simulink model "Battery_Module_Design_Grouped"  (R2021b)
settings: Solver=ode23t  StartTime=0.0  StopTime=36000  MaxStep=0.05  RelTol=1e-3  AbsTol=1e-3
undefined symbols (not defined in the file): batteryCurrent
libraries: fl_lib x5, nesl_utility x4, batteryModule_lib x1
Description:
  | Battery Pack Thermal Management
  | 
  | Copyright 2020-2021 The MathWorks, Inc.
settings Model: Creator=vikrants  LastModifiedBy=smiller
settings SolverCC: AutoScaleAbsTol=off  AlgebraicLoopSolver=TrustRegion
settings DataIOCC: ReturnWorkspaceOutputs=off  SignalLoggingName=logsout_Battery_Module_Design_Grouped
settings DebuggingCC: SymbolicDimsDataTypeCodeGenerationDiagnostic=none  SFMachineParentedDataDiag=warning
settings SFSimCC: CustomCodeUndefinedFunction=UseInterfaceOnly
settings SimscapeCC: SimscapeLogType=all  SimscapeLogSimulationStatistics=on  SimscapeLogName=simlog_Battery_Module_Design_Grouped  SimscapeLogDataHistory=250000

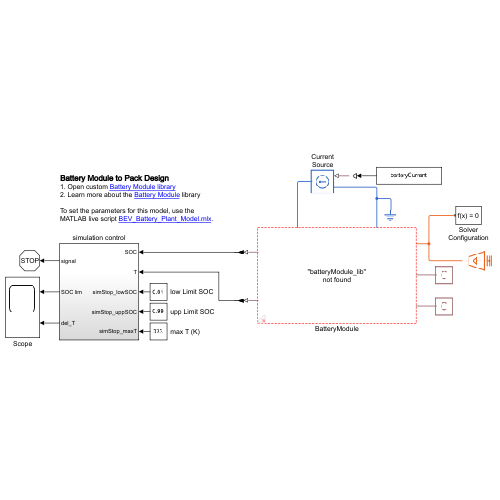
[thumbnail: Simulink's stored preview of the top-level diagram]
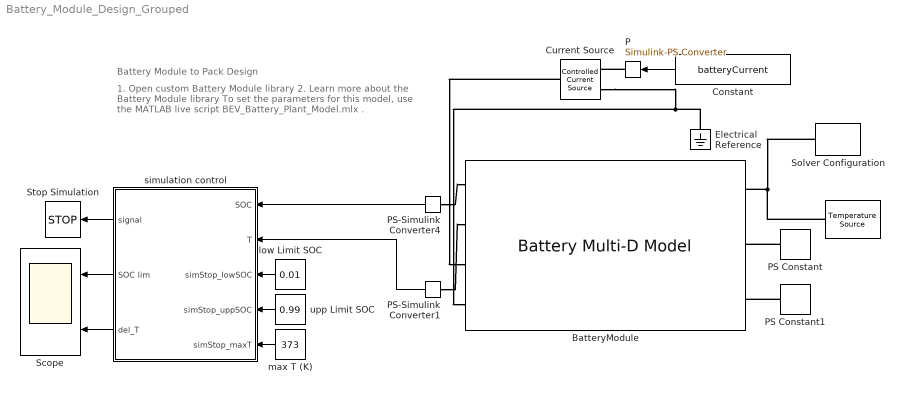
== system Battery_Module_Design_Grouped ==
  note: 1. Open custom Battery Module library
      | 2. Learn more about the Battery Module library
      |
      | To set the parameters for this model, use the
      | MATLAB live script BEV_Battery_Plant_Model.mlx .
  note: Battery Module to Pack Design
  " " : fl_lib/Thermal/Thermal Sources/Temperature Source  temperature=ambientTemp K
  BatteryModule : batteryModule_lib/Battery Multi-D Model  modelComplexity=batteryModule.batteryAbstractionLevel.grouped  thermalManagement=batteryModule.batteryCoolingSystem.thermalPort  thermal_moduleBottom=batteryModule.batteryThermalPortSelection.thermalLUT  thermal_moduleTop=batteryModule.batteryThermalPortSelection.convectionBC  thermal_moduleLeft=batteryModule.batteryThermalPortSelection.convectionBC  thermal_moduleRight=batteryModule.batteryThermalPortSelection.convectionBC  thermal_modulePos=batteryModule.batteryThermalPortSelection.convectionBC  thermal_moduleNeg=batteryModule.batteryThermalPortSelection.convectionBC  Ns=battery_Ns  Np=battery_Np  cellTypeSelection=batteryModule.batteryTypeSelection.pouch  cellHeight=battery_cellH m  cellWidth=battery_cellW m  cellThickness=battery_cellT m  cellDiameter=0.018 m  cellCylinLine=3  moduleExternalR=battery_extR Ohm  LUTpointsTemp=battery_vecT K  LUTpointsSOC=battery_vecSOC  cellAHvector=battery_vecAhr hr*A  moduleCellAHpercentVar=battery_varAhr  cellThermalMass=battery_thermalMass J/K  cellThermalCond=battery_thermalK_thru W/(m*K)  cellThermalCond_inPlane=battery_thermalK_in W/(m*K)  cellHeatTrCoeff=1 W/(m^2 * K)  htc_bottom=1 W/(m^2 * K)  htc_top=battery_sidesHTC W/(m^2 * K)  htc_right=battery_sidesHTC W/(m^2 * K)  htc_left=battery_sidesHTC W/(m^2 * K)  htc_pos=battery_sidesHTC W/(m^2 * K)  htc_neg=battery_sidesHTC W/(m^2 * K)  cellTemp=battery_iniT K  cellSOC=battery_iniSOC  LUTpointsFlowrate_b=vec_coolant_F kg/s  LUTpointsTemp_b=vec_coolant_T K  LUTpointsFlowrate_t=[.01, .02, .03, .04, .05, .06] kg/s  LUTpointsTemp_t=[273.15, 298.15, 323.15] K  LUTpointsFlowrate_r=[.01, .02, .03, .04, .05, .06] kg/s  LUTpointsTemp_r=[273.15, 298.15, 323.15] K  LUTpointsFlowrate_l=[.01, .02, .03, .04, .05, .06] kg/s  LUTpointsTemp_l=[273.15, 298.15, 323.15] K  LUTpointsFlowrate_p=[.01, .02, .03, .04, .05, .06] kg/s  LUTpointsTemp_p=[273.15, 298.15, 323.15] K  LUTpointsFlowrate_n=[.01, .02, .03, .04, .05, .06] kg/s  LUTpointsTemp_n=[273.15, 298.15, 323.15] K  moduleCooling_b=mat_cellQ W/K  moduleCooling_t=zeros(3, 6, 10) W/K  moduleCooling_r=zeros(3, 6, 10) W/K  moduleCooling_l=zeros(3, 6, 10) W/K  moduleCooling_p=zeros(3, 6, 10) W/K  moduleCooling_n=zeros(3, 6, 10) W/K  moduleExtHeat=battery_extHeat W  moduleCellBalancing=batteryModule.batteryCellBalancing.none  passiveShuntR=50 Ohm  passiveSWclosedR=0.01 Ohm  passiveSWopenCond=1e-8 1/Ohm  passiveSWthreshold=0.5  prm_dir=ee.enum.battery.prm_dir.noCurrentDirectionality  V0_mat=battery_V0 V  R0_mat=battery_R0 Ohm  R0_dis_mat=[.03, .015, .002; .04, .017, .008; .039, .012, .006; .027, .013, .021] Ohm  R0_ch_mat=[.03, .015, .002; .04, .017, .008; .039, .012, .006; .027, .013, .021] Ohm  moduleCellR0PercentVar=battery_varR0  prm_leak=ee.enum.battery.prm_leak.disabled  Rleak_vec=[8000, 7000, 6000] Ohm  moduleCellLeakPercentVar=ones(1, 10)  extrapolation_option=ee.enum.extrapolation.nearest  prm_dyn=ee.enum.battery.prm_dyn.rc2  R1_mat=battery_R1 Ohm  tau1_mat=battery_Tau1 s  R2_mat=battery_R2 Ohm  tau2_mat=battery_Tau2 s  R3_mat=[.014, .382, .407; .028, .006, .007; .014, .007, .006; .333, .956, .912] Ohm  tau3_mat=[1, 44, 5644; 11, 24, 506; 2, 14, 330; 3310, 13419, 30216] s  R4_mat=[.014, .382, .407; .028, .006, .007; .014, .007, .006; .333, .956, .912] Ohm  tau4_mat=[1, 44, 5644; 11, 24, 506; 2, 14, 330; 3310, 13419, 30216] s  R5_mat=[.014, .382, .407; .028, .006, .007; .014, .007, .006; .333, .956, .912] Ohm  tau5_mat=[1, 44, 5644; 11, 24, 506; 2, 14, 330; 3310, 13419, 30216] s  prm_fade=ee.enum.battery.prm_fade.equations  N0=100  dV0=0  dR0=0  dAH=0  dRleak=0  dR1=0  dR2=0  dR3=0  dR4=0  dR5=0  N0vec=[100, 200, 300]  Tfadevec=[298.15, 323.15] K  dV0vec=[0, 0, 0]  dR0vec=[0, 0, 0]  dAHvec=[0, 0, 0]  dRleakvec=[0, 0, 0]  dR1vec=[0, 0, 0]  dR2vec=[0, 0, 0]  dR3vec=[0, 0, 0]  dR4vec=[0, 0, 0]  dR5vec=[0, 0, 0]  dV0mat=[0, 0; 0, 0; 0, 0]  dR0mat=[0, 0; 0, 0; 0, 0]  dAHmat=[0, 0; 0, 0; 0, 0]  dRleakmat=[0, 0; 0, 0; 0, 0]  dR1mat=[0, 0; 0, 0; 0, 0]  dR2mat=[0, 0; 0, 0; 0, 0]  dR3mat=[0, 0; 0, 0; 0, 0]  dR4mat=[0, 0; 0, 0; 0, 0]  dR5mat=[0, 0; 0, 0; 0, 0]
      settings: InternalSimscapePortConfiguration="{\"Bottom\":[],\"Left\":[{\"id\":\"outputCellSOC\",\"label\":\"SOC\",\"type\":\"output\"},{\"id\":\"outputCellTemp\",\"label\":\"Temp\",\"type\":\"output\"}],\"Right\":[{\"id\":\"H\",\"label\":\"Amb\",\"type\":\"foundation.thermal.thermal\"},{\"id\":\"frac_b\",\"label\":\"FlwR\",\"type\":\"input\"},{\"id\":\"delT_b\",\"label\":\"FlwT\",\"type\":\"input\"}],\"Top\":[{\"id\":\"p\",\"label\":\"pos\",\"type\":\"foundation.electrical.electrical\"},{\"id\":\"n\",\"label\":\"neg\",\"type\":\"foundation.electrical.electrical\"}]}"
  Constant : Constant  Value=batteryCurrent
  Current Source : fl_lib/Electrical/Electrical Sources/Controlled Current Source
  Electrical Reference : fl_lib/Electrical/Electrical Elements/Electrical Reference
  P : nesl_utility/Simulink-PS Converter  PhysicalDomain=network_engine_domain  SubClassName=ps_input  LeftPortType=input  RightPortType=output  PseudoPeriodic=off  Frequencies=[]  NoiseDistribution=none  NoiseParameters=[]  Unit=A  AffineConversion=off  FilteringAndDerivatives=provide  SimscapeFilterOrder=1  InputFilterTimeConstant=0.001  UdotUserProvided=0
      settings: SourceProductName=Utilities
  PS Constant : fl_lib/Physical Signals/Sources/PS Constant  constant=FlwR
  PS Constant1 : fl_lib/Physical Signals/Sources/PS Constant  constant=FlwT K
  PS-Simulink Converter1 : nesl_utility/PS-Simulink Converter  PhysicalDomain=network_engine_domain  SubClassName=ps_output  LeftPortType=input  RightPortType=output  PseudoPeriodic=off  Frequencies=[]  Unit=K  AffineConversion=on
      settings: SourceProductBaseCode=PW,SS
  PS-Simulink Converter4 : nesl_utility/PS-Simulink Converter  PhysicalDomain=network_engine_domain  SubClassName=ps_output  LeftPortType=input  RightPortType=output  PseudoPeriodic=off  Frequencies=[]  Unit=1  AffineConversion=on
      settings: SourceProductBaseCode=PW,SS
  Scope : Scope  NumInputPorts=2
  Solver Configuration : nesl_utility/Solver Configuration  PhysicalDomain=network_engine_domain  SubClassName=solver  LeftPortType=input  RightPortType=generic  Tones=[]  Harmonics=[]  SimulateNoise=off  Profile=off  UseLocalSampling=off  EnableSwitchedLinearOptims=on  FrequencyDomain=off  UseCCode=off  RelTol=0.001  AbsTol=1e-06  MinStep=1e-09  ToWorkspace=off  RevertToSquareIcSolve=off  NumHomotopyIterations=100  PhasorMode=off  PhasorModeNumHarmonics=1  DoDC=off  ResidualTolerance=1e-09  UseLocalSolver=off  LocalSolverChoice=NE_BACKWARD_EULER_ADVANCER  LocalSolverSampleTime=0.001  DoFixedCost=off  MaxNonlinIter=3  MaxModeIter=2  ComputeImpulses=off  ImpulseIterations=2  LinearAlgebra=auto  EquationFormulation=NE_TIME_EF  DelaysMemoryBudget=1024  AutomaticFiltering=on  FilteringTimeConstant=0.001  PartitionStorageMethod=AS_NEEDED  PartitionMemoryBudget=1024  PartitionMethod=ROBUST
      settings: SourceProductName=Utilities
  Stop Simulation : Stop
  low Limit SOC : Constant  Value=0.01
  max T (K) : Constant  Value=373
  simulation control : Subsystem
  upp Limit SOC : Constant  Value=0.99
  wires:
  Constant/1 -> P/1
  upp Limit SOC/1 -> simulation control/4(simStop_uppSOC)
  low Limit SOC/1 -> simulation control/3(simStop_lowSOC)
  PS-Simulink Converter4/1 -> simulation control/1(SOC)
  max T (K)/1 -> simulation control/5(simStop_maxT)
  simulation control/2(SOC lim) -> Scope/1
  simulation control/3(del_T) -> Scope/2
  simulation control/1(signal) -> Stop Simulation/1
  PS-Simulink Converter1/1 -> simulation control/2(T)
  connections:
  " "/LConn1 -- Solver Configuration/RConn1 -- BatteryModule/RConn1
  Current Source/RConn2 -- Electrical Reference/LConn1 -- BatteryModule/LConn4
  Current Source/LConn1 -- BatteryModule/LConn3
  P/RConn1 -- Current Source/RConn1
  PS-Simulink Converter4/LConn1 -- BatteryModule/LConn1
  PS-Simulink Converter1/LConn1 -- BatteryModule/LConn2
  PS Constant/RConn1 -- BatteryModule/RConn2
  PS Constant1/RConn1 -- BatteryModule/RConn3

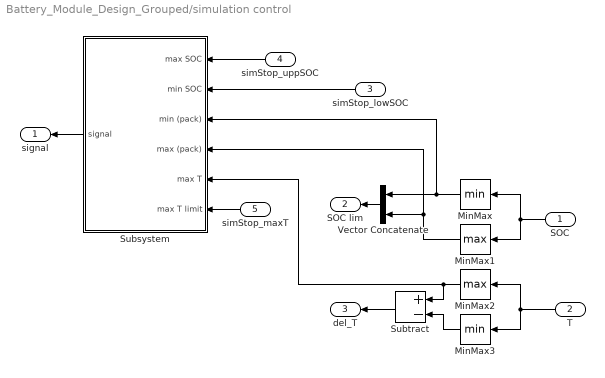
== system Battery_Module_Design_Grouped/simulation control ==
  SOC : Inport
  T : Inport  Port=2
  simStop_lowSOC : Inport  Port=3
  simStop_uppSOC : Inport  Port=4
  simStop_maxT : Inport  Port=5
  MinMax : MinMax
  MinMax1 : MinMax  Function=max
  MinMax2 : MinMax  Function=max
  MinMax3 : MinMax
  Subsystem : Subsystem
  Subtract : Sum  Inputs=+-
  Vector Concatenate : Concatenate
  signal : Outport
  SOC lim : Outport  Port=2
  del_T : Outport  Port=3
  wires:
  MinMax/1 -> Subsystem/3(min (pack)), Vector Concatenate/1
  SOC/1 -> MinMax/1, MinMax1/1
  Vector Concatenate/1 -> SOC lim/1
  MinMax1/1 -> Vector Concatenate/2, Subsystem/4(max (pack))
  T/1 -> MinMax2/1, MinMax3/1
  MinMax2/1 -> Subsystem/5(max T), Subtract/1
  MinMax3/1 -> Subtract/2
  Subtract/1 -> del_T/1
  simStop_maxT/1 -> Subsystem/6(max T limit)
  simStop_uppSOC/1 -> Subsystem/1(max SOC)
  simStop_lowSOC/1 -> Subsystem/2(min SOC)
  Subsystem/1(signal) -> signal/1

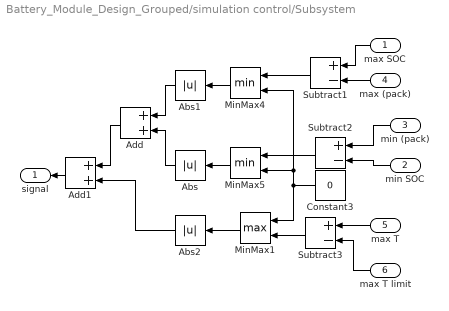
== system Battery_Module_Design_Grouped/simulation control/Subsystem ==
  max SOC : Inport
  min SOC : Inport  Port=2
  min (pack) : Inport  Port=3
  max (pack) : Inport  Port=4
  max T : Inport  Port=5
  max T limit : Inport  Port=6
  Abs : Abs
  Abs1 : Abs
  Abs2 : Abs
  Add : Sum
  Add1 : Sum
  Constant3 : Constant  Value=0
  MinMax1 : MinMax  Function=max  Inputs=2
  MinMax4 : MinMax  Inputs=2
  MinMax5 : MinMax  Inputs=2
  Subtract1 : Sum  Inputs=+-
  Subtract2 : Sum  Inputs=+-
  Subtract3 : Sum  Inputs=+-
  signal : Outport
  wires:
  MinMax5/1 -> Abs/1
  Constant3/1 -> MinMax1/1, MinMax4/2, MinMax5/2
  Abs/1 -> Add/2
  Abs1/1 -> Add/1
  min (pack)/1 -> Subtract2/1
  max SOC/1 -> Subtract1/1
  MinMax4/1 -> Abs1/1
  max (pack)/1 -> Subtract1/2
  min SOC/1 -> Subtract2/2
  Subtract2/1 -> MinMax5/1
  Subtract1/1 -> MinMax4/1
  max T/1 -> Subtract3/1
  max T limit/1 -> Subtract3/2
  Subtract3/1 -> MinMax1/2
  MinMax1/1 -> Abs2/1
  Abs2/1 -> Add1/2
  Add/1 -> Add1/1
  Add1/1 -> signal/1
